simulink model "hip_controller_2026_03_03"  (R2024b)
settings: Solver=FixedStepAuto  StartTime=0.0  StopTime=simDuration  FixedStep=0.01  RelTol=1e-3  EnableMultiTasking=on
InitFcn:
  | breakp=[-1, -0.8, -0.6, -0.4, -0.2, -0.1, 0, 0.1, 0.2, 0.4, 0.6, 0.8, 1];
  | splinenew =[-1, -0.8, -0.6, -0.4, -0.2, -0.1, 0, 0, 0.005, 0.01, 0.015,0.02,0.025];
undefined symbols (not defined in the file or in its folder): Discrete, K, qbreak, Time
libraries: simulink x121, arduinolib x41, dspswit3 x21, ctrlSharedLib x2, dspfdesign x2, slpidlib x2
(part 2 of 7)

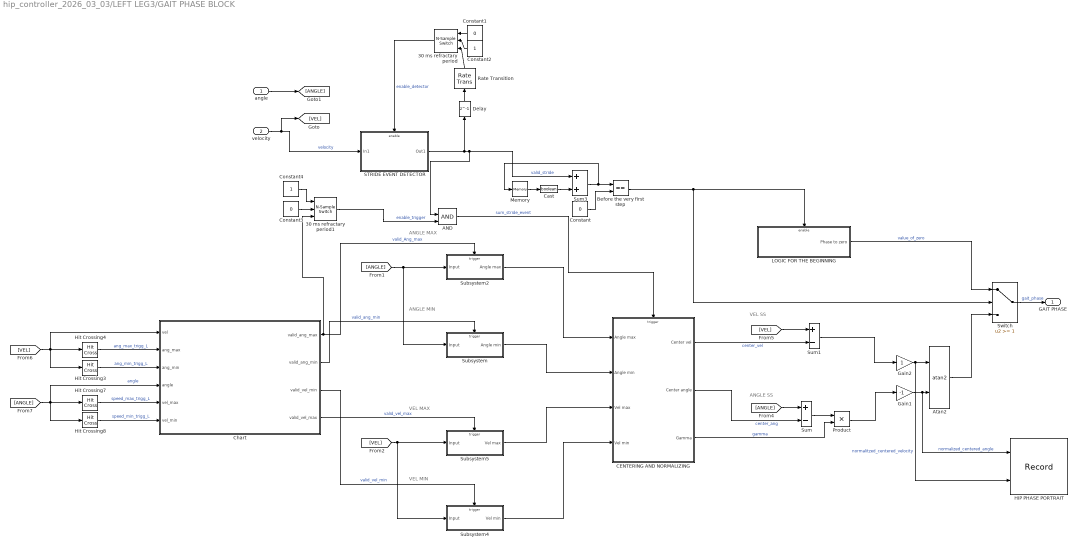
== system hip_controller_2026_03_03/LEFT LEG3/GAIT PHASE BLOCK ==
  note: VEL SS
  note: ANGLE SS
  note: VEL MAX
  note: VEL MIN
  note: ANGLE MIN
  note: ANGLE MAX
  angle : Inport
  velocity : Inport  Port=2
  30 ms refractary period : dspswit3/N-Sample Switch  N=30  reset=on  TriggerType=Rising edge  Ts=-1
  30 ms refractary period1 : dspswit3/N-Sample Switch  N=31  reset=on  TriggerType=Rising edge  Ts=0.01
  AND : Logic  IconShape=distinctive  AllPortsSameDT=off  OutDataTypeStr=boolean
  Atan2 : Trigonometry  Operator=atan2  NumberOfIterations=5
  Before the very first step : RelationalOperator  Operator===  OutDataTypeStr=boolean  RndMeth=Simplest  InputSameDT=off
  CENTERING AND NORMALIZING : Subsystem
  Cast : DataTypeConversion  OutDataTypeStr=boolean  SaturateOnIntegerOverflow=off  RndMeth=Floor
  Chart : Stateflow chart  TreatAsAtomicUnit=on
      settings: PortSchema="{\"entries\":[{\"content\":{\"sides\":[{\"content\":{\"connectorIds\":[\"In5\",\"In1\",\"In4\",\"In6\",\"In3\",\"In2\"]},\"type\":\"ConnectorPlacement.EquallySpacedRectSide\",\"uuid\":\"1b4e9464-0c1b-4aef-9691-eb83c0a92a72\"},{\"content\":{\"connectorIds\":[\"Out3\",\"Out4\",\"Out2\",\"Out1\"],\"side\":\"RIGHT\"},\"type\":\"ConnectorPlacement.EquallySpacedRectSide\",\"uuid\":\"791196f6-4c97-40a1-8015-a03f83b94293\"},{\"content\":{\"side\":\"TOP\"},\"type\":\"ConnectorPlacement.EquallySpacedRectSide\",\"uuid\":\"116d3fb6-be2c-4be4-86cc-df9779b501c6\"}]},\"type\":\"ConnectorPlacement.EquallySpacedConnector\",\"uuid\":\"13d090b2-a2d1-429a-b321-7320a6f027c7\"}],\"packageUris\":[\"http://schema.mathworks.com/mf0/Connector/R2020b\"],\"version\":\"1.0\"}"
  Constant : Constant  Value=0
  Constant1 : Constant  Value=0
  Constant2 : Constant
  Constant3 : Constant  Value=0
  Constant4 : Constant
  Delay : Delay  DelayLength=1
  Gain1 : Gain  Gain=-1
  Gain2 : Gain
  HIP PHASE PORTRAIT : Record  FileSettingsInternal="{\"entries\":[{\"content\":{\"excelSettings\":{\"content\":{},\"type\":\"Streamout.ExcelSettings\"}},\"type\":\"Streamout.FileSettingStorage\",\"uuid\":\"\"}],\"packageUris\":[\"http:\\/\\/schema.mathworks.com\\/mf0\\/streamout_blocks\\/R2020a\"],\"version\":\"1.0\"}"  Layout=[1 1]  SignalsInternal="{\"entries\":[{\"content\":{\"signals\":[{\"content\":{\"blockPath\":[],\"dimensions\":[1],\"domain\":\"\",\"lineColor\":\"#edb120\",\"lineWidth\":2,\"port\":1,\"sid\":[\"\"],\"signalID\":1,\"signalName\":\"normalized_centered_angle\"},\"type\":\"RecordBlkView.Signal\",\"uuid\":\"\"},{\"content\":{\"blockPath\":[],\"dimensions\":[1],\"domain\":\"\",\"lineColor\":\"#7e2f8e\",\"lineWidth\":2,\"port\":2,\"sid\":[\"\"],\"signalID\":2,\"signalName\":\"normalitzed_centered_velocity\"},\"type\":\"RecordBlkView.Signal\",\"uuid\":\"\"}]},\"type\":\"RecordBlkView.InputSignals\",\"uuid\":\"\"}],\"packageUris\":[\"http:\\/\\/schema.mathworks.com\\/mf0\\/streamout_blocks\\/R2020a\"],\"version\":\"1.0\"}"  VisualizationBindings="{\"xyplotplugin\":{\"info\":[{\"series\":[],\"subplotID\":1}]}}"  CompatibilityTag=XY
  Hit Crossing3 : HitCross  HitCrossingDirection=rising
  Hit Crossing4 : HitCross  HitCrossingDirection=falling
  Hit Crossing7 : HitCross  HitCrossingDirection=rising
  Hit Crossing8 : HitCross  HitCrossingDirection=falling
  LOGIC FOR THE BEGINNING : Subsystem
  Memory : Memory
  Product : Product
  Rate Transition : RateTransition  OutPortSampleTime=0.01
  STRIDE EVENT DETECTOR : Subsystem
  Subsystem : Subsystem
  Subsystem2 : Subsystem
  Subsystem4 : Subsystem
  Subsystem5 : Subsystem
  Sum : Sum  Inputs=+-
  Sum1 : Sum  Inputs=+-
  Sum3 : Sum
  Switch : Switch  Threshold=1  SaturateOnIntegerOverflow=off  InputSameDT=off
  GAIT PHASE : Outport
  wires:
  AND/1 -> CENTERING AND NORMALIZING/Trigger  "sum_stride_event"
  Constant4/1 -> 30 ms refractary period1/1
  30 ms refractary period1/1 -> AND/2  "enable_trigger"
  Constant3/1 -> 30 ms refractary period1/2
  Chart/3(valid_ang_max) -> Subsystem2/Trigger, 30 ms refractary period1/3  "valid_Ang_max"
  Chart/1(valid_vel_max) -> Subsystem5/Trigger  "valid_vel_max"
  Chart/2(valid_vel_min) -> Subsystem4/Trigger  "valid_vel_min"
  Chart/4(valid_ang_min) -> Subsystem/Trigger  "valid_ang_min"
  Hit Crossing8/1 -> Chart/2(vel_min)  "speed_min_trigg_L"
  Hit Crossing7/1 -> Chart/3(vel_max)  "speed_max_trigg_L"
  [ANGLE] -> Hit Crossing7/1, Hit Crossing8/1, Chart/6(angle)  "angle"
  Hit Crossing4/1 -> Chart/1(ang_max)  "ang_max_trigg_L"
  Hit Crossing3/1 -> Chart/4(ang_min)  "ang_min_trigg_L"
  [VEL] -> Hit Crossing4/1, Hit Crossing3/1, Chart/5(vel)
  Rate Transition/1 -> 30 ms refractary period/3
  Gain2/1 -> Atan2/1, HIP PHASE PORTRAIT/2  "normalitzed_centered_velocity"
  Delay/1 -> Rate Transition/1
  Constant2/1 -> 30 ms refractary period/2
  Constant1/1 -> 30 ms refractary period/1
  30 ms refractary period/1 -> STRIDE EVENT DETECTOR/Enable  "enable_detector"
  Cast/1 -> Sum3/2
  Memory/1 -> Cast/1
  Switch/1 -> GAIT PHASE/1  "gait_phase"
  LOGIC FOR THE BEGINNING/1(Phase to zero) -> Switch/1  "value_of_zero"
  Before the very first step/1 -> LOGIC FOR THE BEGINNING/Enable, Switch/2
  Constant/1 -> Before the very first step/2
  Sum3/1 -> Before the very first step/1, Memory/1
  Gain1/1 -> Atan2/2, HIP PHASE PORTRAIT/1  "normalized_centered_angle"
  Atan2/1 -> Switch/3
  Sum1/1 -> Gain2/1
  CENTERING AND NORMALIZING/1(Center vel) -> Sum1/2  "center_vel"
  [VEL] -> Sum1/1
  Product/1 -> Gain1/1
  CENTERING AND NORMALIZING/3(Gamma) -> Product/2  "gamma"
  Sum/1 -> Product/1
  CENTERING AND NORMALIZING/2(Center angle) -> Sum/2  "center_ang"
  [ANGLE] -> Sum/1
  Subsystem4/1(Vel min) -> CENTERING AND NORMALIZING/4(Vel min)
  Subsystem5/1(Vel max) -> CENTERING AND NORMALIZING/3(Vel max)
  Subsystem/1(Angle min) -> CENTERING AND NORMALIZING/2(Angle min)
  Subsystem2/1(Angle max) -> CENTERING AND NORMALIZING/1(Angle max)
  STRIDE EVENT DETECTOR/1(Out1) -> Sum3/1, AND/1, Delay/1  "valid_stride"
  [VEL] -> Subsystem5/1(Input), Subsystem4/1(Input)
  [ANGLE] -> Subsystem2/1(Input), Subsystem/1(Input)
  velocity/1 -> [VEL], STRIDE EVENT DETECTOR/1(In1)  "velocity"
  angle/1 -> [ANGLE]

== system hip_controller_2026_03_03/LEFT LEG3/MOTOR POSITION REFERENCE GENERATOR ==
  note: KALMAN FILTER
  GAIT PHASE : Inport
  LAG COMPENSATION : Inport  Port=2
  AMPLITUDE : Inport  Port=3
  Gain : Gain  Gain=-1
  Lookup with Akima spline Interpolation : Lookup_n-D  NumberOfTableDimensions=1  BreakpointsForDimension1=[-5:5]  Table=tanh([-5:5])  InterpMethod=Akima spline  InternalRulePriority=Speed  RndMeth=Simplest
  Motion mapping2 : Lookup_n-D  NumberOfTableDimensions=1  BreakpointsForDimension1=[-1, -0.8, -0.6, -0.4, -0.2, -0.1, 0, 0.1, 0.2, 0.4, 0.6, 0.8, 1]  BreakpointsForDimension2=qbreak(:,2)  Table=[-1, -0.8, -0.6, -0.4, -0.2, -0.1, 0, 0, 0.005, 0.01, 0.015,0.02,0.025]  InterpMethod=Cubic spline  ExtrapMethod=Cubic spline  InternalRulePriority=Speed  RndMeth=Simplest
  Plus : Sum
  Product : Product
  Product1 : Product
  Rate Transition : RateTransition  OutPortSampleTime=0.01
  Ref traj w/ noise : ctrlSharedLib/Kalman Filter  Commented=on  TimeDomain=Discrete-Time  UseCurrentEstimator=off  ModelSource=Individual A, B, C, D matrices  ModelSourceVariable=ss(0.95,1,1,0,1)  A=[1]  B=1  C=[1]  D=0  NumberOfStates=1  NumberOfInputs=1  NumberOfOutputs=1  InitialEstimateSource=Dialog  X0=[0]  P0=10  UseK=off  UseGH=off  NumberOfProcessNoiseInputs=1  G=1  TimeInvariantG=on  H=0  TimeInvariantH=on  Q=1e-3  TimeInvariantQ=on  R=9e-4  TimeInvariantR=on  N=0  TimeInvariantN=on  AddInputPort=off  AddEnablePort=off  OutputEstimatedY=off  OutputP=off  Ts=-1
  Saturation : Saturate  UpperLimit=600*pi/180  LowerLimit=-600*pi/180
  Sin1 : Trigonometry
  Ref motion : Outport
  wires:
  Rate Transition/1 -> Motion mapping2/1  "motion_mapping_key"
  Saturation/1 -> Ref motion/1  "reference_motion"
  Gain/1 -> Rate Transition/1  "left_sin_wave"
  AMPLITUDE/1 -> Product/2  "amplitude"
  LAG COMPENSATION/1 -> Plus/2
  GAIT PHASE/1 -> Plus/1  "gait_phase_left"
  Plus/1 -> Sin1/1
  Sin1/1 -> Gain/1
  Product/1 -> Saturation/1
  Motion mapping2/1 -> Product/1  "motion_mapping_value"
  ? -> Product1/2
  ? -> Product1/1  "motion_mapping_value"

== system hip_controller_2026_03_03/LEFT LEG3/Subsystem ==
  Angle estimation : Inport
  Velocity surrogate (quarature component) : Inport  Port=2
  classif : Inport  Port=3
  Ref amplitude : Inport  Port=4
  sig_power : Inport  Port=5
  Cast To Double : DataTypeConversion  OutDataTypeStr=double  SaturateOnIntegerOverflow=off  RndMeth=Floor
  Chart1 : Stateflow chart  TreatAsAtomicUnit=on
  Constant : Constant
  Product : Product
  Product1 : Product
  SIGMOID SCALING : Subsystem
  Sqrt : Sqrt
  Square : Math  Operator=square
  Square1 : Math  Operator=square
  Sum : Sum
  AMPLITUDE : Outport
  wires:
  Constant/1 -> Chart1/4(Scale_LM)
  Chart1/1(scale) -> Product1/2  "scale=1"
  Product1/1 -> SIGMOID SCALING/1(PORTRAIT RADIUS)
  Angle estimation/1 -> Square/1
  Ref amplitude/1 -> Chart1/2(amplitude)
  sig_power/1 -> Chart1/3(sig_power)
  Velocity surrogate (quarature component)/1 -> Square1/1
  Chart1/2(gain) -> Product/2  "gain=amplitude=6.5"
  Chart1/3(sigmoid_power) -> SIGMOID SCALING/2(Sigmoid Power)  "sigmoid_power=50"
  classif/1 -> Cast To Double/1
  Cast To Double/1 -> Chart1/1(class)
  SIGMOID SCALING/1(Out1) -> Product/1
  Sqrt/1 -> Product1/1  "PORTRAIT RADIUS"
  Product/1 -> AMPLITUDE/1
  Sum/1 -> Sqrt/1
  Square1/1 -> Sum/2
  Square/1 -> Sum/1

== system hip_controller_2026_03_03/Prerecorded Data/Subsystem1 ==
  x : Inport
  Constant : Constant  Value=2
  Integrator1 : Integrator  InitialConditionSource=external
  Integrator2 : Integrator
  Product : Product  RndMeth=Zero
  Product1 : Product  RndMeth=Zero
  Product2 : Product  Inputs=3  RndMeth=Zero
  Sum : Sum  Inputs=|+-
  Sum1 : Sum  Inputs=|+-
  wn : Constant  Value=wn
  x0 : Constant  Value=x0
  zt : Constant  Value=zt
  y : Outport  VectorParamsAs1DForOutWhenUnconnected=off
  wires:
  Sum/1 -> Product/2
  wn/1 -> Product/1, Product1/1
  Sum1/1 -> Sum/1
  x0/1 -> Integrator1/2
  Integrator2/1 -> Product1/2, Product2/1
  Product/1 -> Integrator2/1
  x/1 -> Sum1/1
  Product1/1 -> Integrator1/1
  Integrator1/1 -> Sum1/2, y/1
  Product2/1 -> Sum/2
  zt/1 -> Product2/3
  Constant/1 -> Product2/2

== system hip_controller_2026_03_03/Prerecorded Data/Subsystem2 ==
  x : Inport
  Constant : Constant  Value=2
  Integrator1 : Integrator  InitialConditionSource=external
  Integrator2 : Integrator
  Product : Product  RndMeth=Zero
  Product1 : Product  RndMeth=Zero
  Product2 : Product  Inputs=3  RndMeth=Zero
  Sum : Sum  Inputs=|+-
  Sum1 : Sum  Inputs=|+-
  wn : Constant  Value=wn
  x0 : Constant  Value=x0
  zt : Constant  Value=zt
  y : Outport  VectorParamsAs1DForOutWhenUnconnected=off
  yd : Outport  Port=2
  wires:
  Sum/1 -> Product/2  "e2=e1-feedback"
  wn/1 -> Product/1, Product1/1  "wn"
  Sum1/1 -> Sum/1  "e1=x-y"
  x0/1 -> Integrator1/2  "x0=0"
  Integrator2/1 -> Product2/1, Product1/2  "integrator(wn*e2)"
  Product/1 -> Integrator2/1  "wn*e2"
  x/1 -> Sum1/1  "x"
  Product1/1 -> Integrator1/1, yd/1  "yd"
  Integrator1/1 -> Sum1/2, y/1  "y"
  Product2/1 -> Sum/2  "feedback"
  zt/1 -> Product2/3  "zt=1"
  Constant/1 -> Product2/2

== system hip_controller_2026_03_03/Prerecorded Data/Subsystem3 ==
  x : Inport
  Constant : Constant  Value=2
  Integrator1 : Integrator  InitialConditionSource=external
  Integrator2 : Integrator
  Product : Product  RndMeth=Zero
  Product1 : Product  RndMeth=Zero
  Product2 : Product  Inputs=3  RndMeth=Zero
  Sum : Sum  Inputs=|+-
  Sum1 : Sum  Inputs=|+-
  wn : Constant  Value=wn
  x0 : Constant  Value=x0
  zt : Constant  Value=zt
  y : Outport  VectorParamsAs1DForOutWhenUnconnected=off
  wires:
  Sum/1 -> Product/2
  wn/1 -> Product/1, Product1/1
  Sum1/1 -> Sum/1
  x0/1 -> Integrator1/2
  Integrator2/1 -> Product1/2, Product2/1
  Product/1 -> Integrator2/1
  x/1 -> Sum1/1
  Product1/1 -> Integrator1/1
  Integrator1/1 -> Sum1/2, y/1
  Product2/1 -> Sum/2
  zt/1 -> Product2/3
  Constant/1 -> Product2/2

== system hip_controller_2026_03_03/Prerecorded Data/Subsystem4 ==
  x : Inport
  Constant : Constant  Value=2
  Integrator1 : Integrator  InitialConditionSource=external
  Integrator2 : Integrator
  Product : Product  RndMeth=Zero
  Product1 : Product  RndMeth=Zero
  Product2 : Product  Inputs=3  RndMeth=Zero
  Sum : Sum  Inputs=|+-
  Sum1 : Sum  Inputs=|+-
  wn : Constant  Value=wn
  x0 : Constant  Value=x0
  zt : Constant  Value=zt
  y : Outport  VectorParamsAs1DForOutWhenUnconnected=off
  wires:
  Sum/1 -> Product/2
  wn/1 -> Product/1, Product1/1
  Sum1/1 -> Sum/1
  x0/1 -> Integrator1/2
  Integrator2/1 -> Product1/2, Product2/1
  Product/1 -> Integrator2/1
  x/1 -> Sum1/1
  Product1/1 -> Integrator1/1
  Integrator1/1 -> Sum1/2, y/1
  Product2/1 -> Sum/2
  zt/1 -> Product2/3
  Constant/1 -> Product2/2

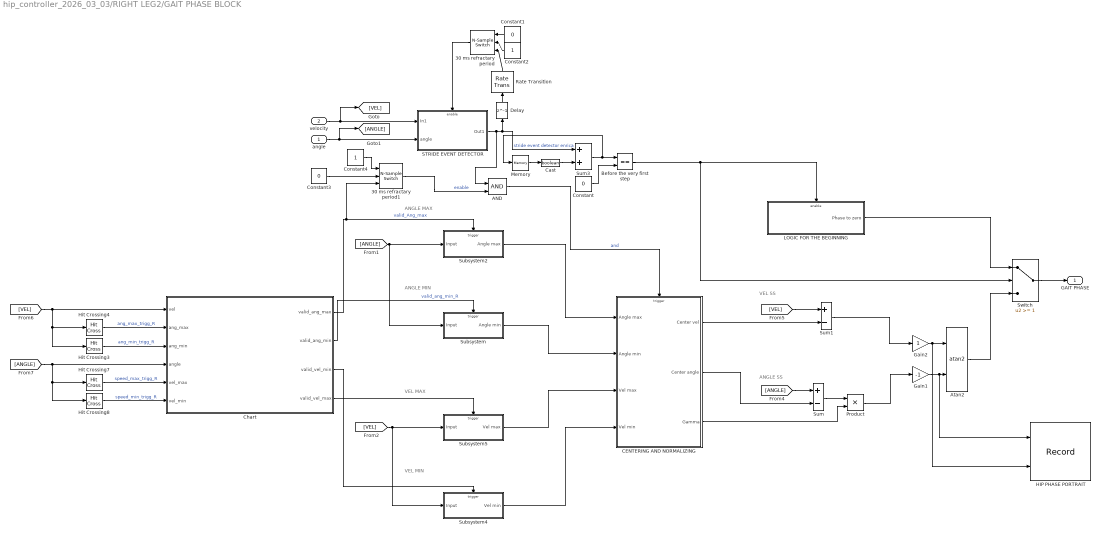
== system hip_controller_2026_03_03/RIGHT LEG2/GAIT PHASE BLOCK ==
  note: VEL SS
  note: ANGLE SS
  note: VEL MAX
  note: VEL MIN
  note: ANGLE MIN
  note: ANGLE MAX
  angle : Inport
  velocity : Inport  Port=2
  30 ms refractary period : dspswit3/N-Sample Switch  N=30  reset=on  TriggerType=Rising edge  Ts=-1
  30 ms refractary period1 : dspswit3/N-Sample Switch  N=31  reset=on  TriggerType=Rising edge  Ts=0.01
  AND : Logic  IconShape=distinctive  AllPortsSameDT=off  OutDataTypeStr=boolean
  Atan2 : Trigonometry  Operator=atan2  NumberOfIterations=5
  Before the very first step : RelationalOperator  Operator===  OutDataTypeStr=boolean  RndMeth=Simplest  InputSameDT=off
  CENTERING AND NORMALIZING : Subsystem
  Cast : DataTypeConversion  OutDataTypeStr=boolean  SaturateOnIntegerOverflow=off  RndMeth=Floor
  Chart : Stateflow chart  TreatAsAtomicUnit=on
      settings: PortSchema="{\"entries\":[{\"content\":{\"sides\":[{\"content\":{\"connectorIds\":[\"In5\",\"In1\",\"In4\",\"In6\",\"In3\",\"In2\"]},\"type\":\"ConnectorPlacement.EquallySpacedRectSide\",\"uuid\":\"1b4e9464-0c1b-4aef-9691-eb83c0a92a72\"},{\"content\":{\"connectorIds\":[\"Out3\",\"Out4\",\"Out2\",\"Out1\"],\"side\":\"RIGHT\"},\"type\":\"ConnectorPlacement.EquallySpacedRectSide\",\"uuid\":\"791196f6-4c97-40a1-8015-a03f83b94293\"},{\"content\":{\"side\":\"TOP\"},\"type\":\"ConnectorPlacement.EquallySpacedRectSide\",\"uuid\":\"116d3fb6-be2c-4be4-86cc-df9779b501c6\"}]},\"type\":\"ConnectorPlacement.EquallySpacedConnector\",\"uuid\":\"13d090b2-a2d1-429a-b321-7320a6f027c7\"}],\"packageUris\":[\"http://schema.mathworks.com/mf0/Connector/R2020b\"],\"version\":\"1.0\"}"
  Constant : Constant  Value=0
  Constant1 : Constant  Value=0
  Constant2 : Constant
  Constant3 : Constant  Value=0
  Constant4 : Constant
  Delay : Delay  DelayLength=1
  Gain1 : Gain  Gain=-1
  Gain2 : Gain
  HIP PHASE PORTRAIT : Record  FileSettingsInternal="{\"entries\":[{\"content\":{\"excelSettings\":{\"content\":{},\"type\":\"Streamout.ExcelSettings\"}},\"type\":\"Streamout.FileSettingStorage\",\"uuid\":\"\"}],\"packageUris\":[\"http:\\/\\/schema.mathworks.com\\/mf0\\/streamout_blocks\\/R2020a\"],\"version\":\"1.0\"}"  Layout=[1 1]  SignalsInternal="{\"entries\":[{\"content\":{\"signals\":[{\"content\":{\"blockPath\":[],\"dimensions\":[1],\"domain\":\"\",\"lineColor\":\"#ff6929\",\"lineWidth\":2,\"port\":1,\"sid\":[\"\"],\"signalID\":1,\"signalName\":\"Gain1\"},\"type\":\"RecordBlkView.Signal\",\"uuid\":\"\"},{\"content\":{\"blockPath\":[],\"dimensions\":[1],\"domain\":\"\",\"lineColor\":\"#b746ff\",\"lineWidth\":2,\"port\":2,\"sid\":[\"\"],\"signalID\":2,\"signalName\":\"Gain2\"},\"type\":\"RecordBlkView.Signal\",\"uuid\":\"\"}]},\"type\":\"RecordBlkView.InputSignals\",\"uuid\":\"\"}],\"packageUris\":[\"http:\\/\\/schema.mathworks.com\\/mf0\\/streamout_blocks\\/R2020a\"],\"version\":\"1.0\"}"  VisualizationBindings="{\"xyplotplugin\":{\"info\":[{\"series\":[],\"subplotID\":1}]}}"  CompatibilityTag=XY
  Hit Crossing3 : HitCross  HitCrossingDirection=rising
  Hit Crossing4 : HitCross  HitCrossingDirection=falling
  Hit Crossing7 : HitCross  HitCrossingDirection=rising
  Hit Crossing8 : HitCross  HitCrossingDirection=falling
  LOGIC FOR THE BEGINNING : Subsystem
  Memory : Memory
  Product : Product
  Rate Transition : RateTransition  OutPortSampleTime=0.01
  STRIDE EVENT DETECTOR : Subsystem
  Subsystem : Subsystem
  Subsystem2 : Subsystem
  Subsystem4 : Subsystem
  Subsystem5 : Subsystem
  Sum : Sum  Inputs=+-
  Sum1 : Sum  Inputs=+-
  Sum3 : Sum
  Switch : Switch  Threshold=1  SaturateOnIntegerOverflow=off  InputSameDT=off
  GAIT PHASE : Outport
  wires:
  AND/1 -> CENTERING AND NORMALIZING/Trigger  "and"
  Constant4/1 -> 30 ms refractary period1/1
  STRIDE EVENT DETECTOR/1(Out1) -> Sum3/1, Delay/1, AND/1  "stride event detector enrica"
  30 ms refractary period1/1 -> AND/2  "enable"
  Constant3/1 -> 30 ms refractary period1/2
  Chart/3(valid_ang_max) -> 30 ms refractary period1/3, Subsystem2/Trigger  "valid_Ang_max"
  Chart/1(valid_vel_max) -> Subsystem5/Trigger
  Chart/4(valid_ang_min) -> Subsystem/Trigger  "valid_ang_min_R"
  Hit Crossing8/1 -> Chart/2(vel_min)  "speed_min_trigg_R"
  Hit Crossing4/1 -> Chart/1(ang_max)  "ang_max_trigg_R"
  [ANGLE] -> Chart/6(angle), Hit Crossing7/1, Hit Crossing8/1
  Hit Crossing7/1 -> Chart/3(vel_max)  "speed_max_trigg_R"
  [VEL] -> Chart/5(vel), Hit Crossing4/1, Hit Crossing3/1
  Hit Crossing3/1 -> Chart/4(ang_min)  "ang_min_trigg_R"
  Rate Transition/1 -> 30 ms refractary period/3
  Gain2/1 -> Atan2/1, HIP PHASE PORTRAIT/2
  Delay/1 -> Rate Transition/1
  Constant2/1 -> 30 ms refractary period/2
  Constant1/1 -> 30 ms refractary period/1
  30 ms refractary period/1 -> STRIDE EVENT DETECTOR/Enable
  Cast/1 -> Sum3/2
  Memory/1 -> Cast/1
  Switch/1 -> GAIT PHASE/1
  LOGIC FOR THE BEGINNING/1(Phase to zero) -> Switch/1
  Before the very first step/1 -> LOGIC FOR THE BEGINNING/Enable, Switch/2
  Constant/1 -> Before the very first step/2
  Sum3/1 -> Before the very first step/1, Memory/1
  Gain1/1 -> Atan2/2, HIP PHASE PORTRAIT/1
  Atan2/1 -> Switch/3
  Sum1/1 -> Gain2/1
  CENTERING AND NORMALIZING/1(Center vel) -> Sum1/2
  [VEL] -> Sum1/1
  Product/1 -> Gain1/1
  CENTERING AND NORMALIZING/3(Gamma) -> Product/2
  Sum/1 -> Product/1
  CENTERING AND NORMALIZING/2(Center angle) -> Sum/2
  [ANGLE] -> Sum/1
  Subsystem4/1(Vel min) -> CENTERING AND NORMALIZING/4(Vel min)
  Subsystem5/1(Vel max) -> CENTERING AND NORMALIZING/3(Vel max)
  Subsystem/1(Angle min) -> CENTERING AND NORMALIZING/2(Angle min)
  Subsystem2/1(Angle max) -> CENTERING AND NORMALIZING/1(Angle max)
  [VEL] -> Subsystem5/1(Input), Subsystem4/1(Input)
  Chart/2(valid_vel_min) -> Subsystem4/Trigger
  [ANGLE] -> Subsystem2/1(Input), Subsystem/1(Input)
  velocity/1 -> [VEL], STRIDE EVENT DETECTOR/1(In1)
  angle/1 -> STRIDE EVENT DETECTOR/2(angle), [ANGLE]

== system hip_controller_2026_03_03/RIGHT LEG2/MOTOR POSITION REFERENCE GENERATOR ==
  note: KALMAN FILTER
  GAIT PHASE : Inport
  LAG COMPENSATION : Inport  Port=2
  AMPLITUDE : Inport  Port=3
  Gain : Gain  Gain=-1
  Motion mapping2 : Lookup_n-D  NumberOfTableDimensions=1  BreakpointsForDimension1=[-1, -0.8, -0.6, -0.4, -0.2, -0.1, 0, 0.1, 0.2, 0.4, 0.6, 0.8, 1]  BreakpointsForDimension2=qbreak(:,2)  Table=[-1, -0.8, -0.6, -0.4, -0.2, -0.1, 0, 0, 0.005, 0.01, 0.015,0.02,0.025]  InterpMethod=Cubic spline  ExtrapMethod=Cubic spline  InternalRulePriority=Speed  RndMeth=Simplest
  Plus : Sum
  Product : Product
  Rate Transition : RateTransition  OutPortSampleTime=0.01
  Ref traj w/ noise : ctrlSharedLib/Kalman Filter  Commented=on  TimeDomain=Discrete-Time  UseCurrentEstimator=off  ModelSource=Individual A, B, C, D matrices  ModelSourceVariable=ss(0.95,1,1,0,1)  A=[1]  B=1  C=[1]  D=0  NumberOfStates=1  NumberOfInputs=1  NumberOfOutputs=1  InitialEstimateSource=Dialog  X0=[0]  P0=10  UseK=off  UseGH=off  NumberOfProcessNoiseInputs=1  G=1  TimeInvariantG=on  H=0  TimeInvariantH=on  Q=1e-3  TimeInvariantQ=on  R=9e-4  TimeInvariantR=on  N=0  TimeInvariantN=on  AddInputPort=off  AddEnablePort=off  OutputEstimatedY=off  OutputP=off  Ts=-1
  Saturation : Saturate  UpperLimit=600*pi/180  LowerLimit=-600*pi/180
  Sin1 : Trigonometry
  Ref motion : Outport
  wires:
  Rate Transition/1 -> Motion mapping2/1  "right_sin_wave"
  Saturation/1 -> Ref motion/1  "ref_motion"
  Gain/1 -> Rate Transition/1  "sin_wave"
  AMPLITUDE/1 -> Product/2  "amplitude"
  LAG COMPENSATION/1 -> Plus/2
  GAIT PHASE/1 -> Plus/1  "gait_phase"
  Plus/1 -> Sin1/1
  Sin1/1 -> Gain/1
  Product/1 -> Saturation/1
  Motion mapping2/1 -> Product/1

== system hip_controller_2026_03_03/RIGHT LEG2/Subsystem ==
  Angle estimation : Inport
  Velocity surrogate (quarature component) : Inport  Port=2
  Ref amplitude : Inport  Port=3
  classif : Inport  Port=4
  Sig_Power : Inport  Port=5
  Cast To Double : DataTypeConversion  OutDataTypeStr=double  SaturateOnIntegerOverflow=off  RndMeth=Floor
  Chart1 : Stateflow chart  TreatAsAtomicUnit=on
  Constant : Constant
  Product : Product
  Product1 : Product
  SIGMOID SCALING : Subsystem
  Sqrt : Sqrt
  Square : Math  Operator=square
  Square1 : Math  Operator=square
  Sum : Sum
  Amplitude_R : Outport
  wires:
  Chart1/1(scale_LM) -> Product1/2
  Constant/1 -> Chart1/4("scale_LM "), Chart1/5(Scale)
  Product1/1 -> SIGMOID SCALING/1(PORTRAIT RADIUS)
  Angle estimation/1 -> Square/1
  Sig_Power/1 -> Chart1/3(sig_power)
  Velocity surrogate (quarature component)/1 -> Square1/1
  Chart1/2(gain) -> Product/2
  Sqrt/1 -> Product1/1  "PORTRAIT RADIUS R"
  Chart1/3(sigmoid_power) -> SIGMOID SCALING/2(sigmoid_power)
  Ref amplitude/1 -> Chart1/2(amplitude)
  classif/1 -> Cast To Double/1
  Cast To Double/1 -> Chart1/1(class)
  SIGMOID SCALING/1(Out1) -> Product/1  "Sig_Scale_R"
  Product/1 -> Amplitude_R/1
  Sum/1 -> Sqrt/1
  Square1/1 -> Sum/2
  Square/1 -> Sum/1

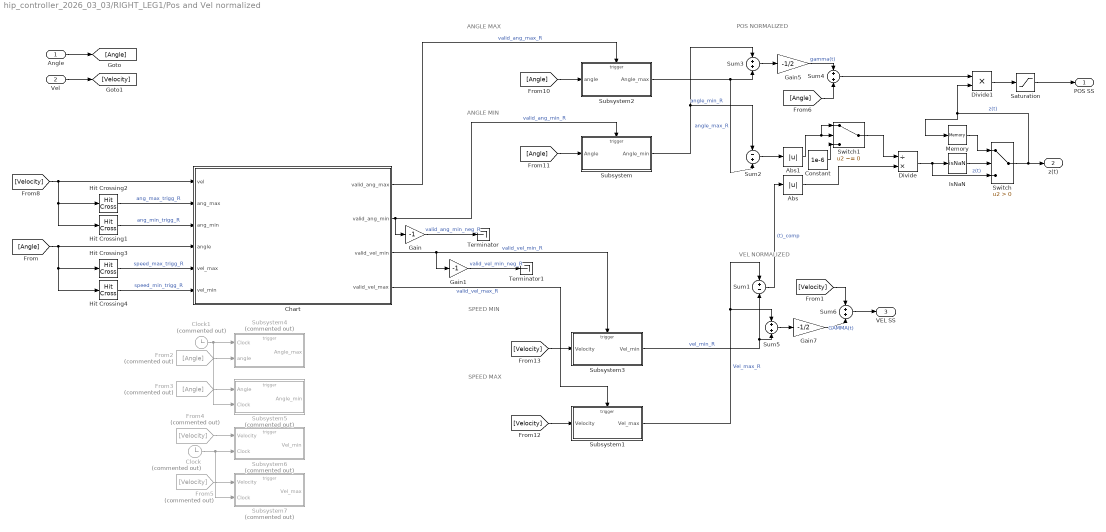
== system hip_controller_2026_03_03/RIGHT_LEG1/Pos and Vel normalized ==
  note: ANGLE MIN
  note: ANGLE MAX
  note: SPEED MAX
  note: SPEED MIN
  note: POS NORMALIZED
  note: VEL NORMALIZED
  Angle : Inport
  Vel : Inport  Port=2
  Abs : Abs  SaturateOnIntegerOverflow=off
  Abs1 : Abs  SaturateOnIntegerOverflow=off
  Chart : Stateflow chart  TreatAsAtomicUnit=on
      settings: PortSchema="{\"entries\":[{\"content\":{\"sides\":[{\"content\":{\"connectorIds\":[\"In5\",\"In1\",\"In4\",\"In6\",\"In3\",\"In2\"]},\"type\":\"ConnectorPlacement.EquallySpacedRectSide\",\"uuid\":\"1b4e9464-0c1b-4aef-9691-eb83c0a92a72\"},{\"content\":{\"connectorIds\":[\"Out3\",\"Out4\",\"Out2\",\"Out1\"],\"side\":\"RIGHT\"},\"type\":\"ConnectorPlacement.EquallySpacedRectSide\",\"uuid\":\"791196f6-4c97-40a1-8015-a03f83b94293\"},{\"content\":{\"side\":\"TOP\"},\"type\":\"ConnectorPlacement.EquallySpacedRectSide\",\"uuid\":\"116d3fb6-be2c-4be4-86cc-df9779b501c6\"}]},\"type\":\"ConnectorPlacement.EquallySpacedConnector\",\"uuid\":\"13d090b2-a2d1-429a-b321-7320a6f027c7\"}],\"packageUris\":[\"http://schema.mathworks.com/mf0/Connector/R2020b\"],\"version\":\"1.0\"}"
  Clock : Clock  Commented=on
  Clock1 : Clock  Commented=on
  Constant : Constant  Value=1e-6
  Divide : Product  Inputs=/*
  Divide1 : Product  Inputs=**
  From2 : From  Commented=on  GotoTag=Angle
  From3 : From  Commented=on  GotoTag=Angle
  From4 : From  Commented=on  GotoTag=Velocity
  From5 : From  Commented=on  GotoTag=Velocity
  Gain : Gain  Gain=-1
  Gain1 : Gain  Gain=-1
  Gain5 : Gain  Gain=-1/2
  Gain7 : Gain  Gain=-1/2
  Hit Crossing1 : HitCross  HitCrossingDirection=rising
  Hit Crossing2 : HitCross  HitCrossingDirection=falling
  Hit Crossing3 : HitCross  HitCrossingDirection=rising
  Hit Crossing4 : HitCross  HitCrossingDirection=falling
  IsNaN : RelationalOperator  Operator=isNaN  OutDataTypeStr=boolean  RndMeth=Simplest  InputSameDT=off
  Memory : Memory
  Saturation : Saturate  UpperLimit=10  LowerLimit=-10
  Subsystem : Subsystem
  Subsystem1 : Subsystem
  Subsystem2 : Subsystem
  Subsystem3 : Subsystem
  Subsystem4 : Subsystem  Commented=on
  Subsystem5 : Subsystem  Commented=on
  Subsystem6 : Subsystem  Commented=on
  Subsystem7 : Subsystem  Commented=on
  Sum1 : Sum  Inputs=+-
  Sum2 : Sum  Inputs=-+
  Sum{3..6} (4 alike) : Sum
  Switch : Switch  Criteria=u2 > Threshold  SaturateOnIntegerOverflow=off  InputSameDT=off
  Switch1 : Switch  Criteria=u2 ~= 0  SaturateOnIntegerOverflow=off  InputSameDT=off
  Terminator : Terminator
  Terminator1 : Terminator
  POS SS : Outport
  z(t) : Outport  Port=2
  VEL SS : Outport  Port=3
  wires:
  Hit Crossing2/1 -> Chart/1(ang_max)  "ang_max_trigg_R"
  Subsystem2/1(Angle_max) -> Sum2/2, Sum3/2  "angle_max_R"
  Sum4/1 -> Divide1/1
  Sum3/1 -> Gain5/1
  Subsystem/1(Angle_min) -> Sum2/1, Sum3/1  "angle_min_R"
  Hit Crossing1/1 -> Chart/4(ang_min)  "ang_min_trigg_R"
  Sum2/1 -> Abs1/1
  Sum1/1 -> Abs/1  "(t)_comp"
  Gain5/1 -> Sum4/1  "gamma(t)"
  Abs/1 -> Divide/2
  Divide/1 -> IsNaN/1, Switch/3  "z(t)"
  Memory/1 -> Switch/1
  IsNaN/1 -> Switch/2
  Switch/1 -> Memory/1, Divide1/2, z(t)/1  "z(t)"
  Divide1/1 -> Saturation/1
  Saturation/1 -> POS SS/1
  Clock1/1 -> Subsystem5/2(Clock), Subsystem4/1(Clock)
  Constant/1 -> Switch1/3
  Abs1/1 -> Switch1/2, Switch1/1
  Switch1/1 -> Divide/1
  Clock/1 -> Subsystem7/2(Clock), Subsystem6/2(Clock)
  Hit Crossing4/1 -> Chart/2(vel_min)  "speed_min_trigg_R"
  Subsystem3/1(Vel_min) -> Sum1/2, Sum5/2  "vel_min_R"
  Subsystem1/1(Vel_max) -> Sum1/1, Sum5/1  "Vel_max_R"
  Sum5/1 -> Gain7/1
  Hit Crossing3/1 -> Chart/3(vel_max)  "speed_max_trigg_R"
  Sum6/1 -> VEL SS/1
  Gain7/1 -> Sum6/2  "GAMMA(t)"
  [Velocity] -> Sum6/1
  Chart/1(valid_vel_max) -> Subsystem1/Trigger  "valid_vel_max_R"
  Chart/4(valid_ang_min) -> Gain/1, Subsystem/Trigger  "valid_ang_min_R"
  Chart/3(valid_ang_max) -> Subsystem2/Trigger  "valid_ang_max_R"
  Chart/2(valid_vel_min) -> Gain1/1, Subsystem3/Trigger  "valid_vel_min_R"
  Vel/1 -> [Velocity]
  Angle/1 -> [Angle]
  From5/1 -> Subsystem7/1(Velocity)
  From4/1 -> Subsystem6/1(Velocity)
  From3/1 -> Subsystem5/1(Angle)
  From2/1 -> Subsystem4/2(angle)
  [Angle] -> Hit Crossing4/1, Hit Crossing3/1, Chart/6(angle)
  [Angle] -> Subsystem/1(Angle)
  [Angle] -> Subsystem2/1(angle)
  [Velocity] -> Subsystem1/1(Velocity)
  [Velocity] -> Subsystem3/1(Velocity)
  [Velocity] -> Hit Crossing1/1, Hit Crossing2/1, Chart/5(vel)
  Gain/1 -> Terminator/1  "valid_ang_min_neg_R"
  Gain1/1 -> Terminator1/1  "valid_vel_min_neg_R"
  [Angle] -> Sum4/2

== system hip_controller_2026_03_03/RIGHT_LEG1/STOP CONDITION ==
  position : Inport
  speed : Inport  Port=2
  Constant : Constant
  Constant1 : Constant  Value=0
  Sqrt : Sqrt
  Square : Math  Operator=square
  Square1 : Math  Operator=square
  Sum : Sum
  Switch3 : Switch  Criteria=u2 > Threshold  Threshold=0.3  SaturateOnIntegerOverflow=off  InputSameDT=off
  Check : Outport
  Walking frequency : Outport  Port=2
  wires:
  position/1 -> Square/1  "θ"
  speed/1 -> Square1/1  "θ_dot"
  Square/1 -> Sum/1
  Square1/1 -> Sum/2
  Sum/1 -> Sqrt/1
  Constant/1 -> Switch3/1
  Constant1/1 -> Switch3/3
  Sqrt/1 -> Switch3/2, Walking frequency/1
  Switch3/1 -> Check/1

== system hip_controller_2026_03_03/Subsystem3/Left Motor Velocity ==
  SWITCH : Inport
  Motor command : Inport  Port=2
  Motor Actual Position Receive : Subsystem
  Subsystem : Subsystem
  MOTOR POSITION : Outport
  MOTOR SPEED : Outport  Port=2
  MOTOR TORQUE : Outport  Port=3
  wires:
  Motor command/1 -> Subsystem/1(Motor command)
  SWITCH/1 -> Motor Actual Position Receive/1(SWITCH), Subsystem/2(SWITCH)
  Motor Actual Position Receive/1(MOTOR POSITION) -> MOTOR POSITION/1
  Motor Actual Position Receive/2(MOTOR SPEED) -> MOTOR SPEED/1
  Motor Actual Position Receive/3(MOTOR TORQUE) -> MOTOR TORQUE/1

== system hip_controller_2026_03_03/Subsystem3/Right Motor Velocity ==
  SWITCH : Inport
  Motor command : Inport  Port=2
  Motor Actual Position Receive : Subsystem
  Subsystem : Subsystem
  MOTOR POSITION : Outport
  MOTOR SPEED : Outport  Port=2
  MOTOR TORQUE : Outport  Port=3
  wires:
  Motor command/1 -> Subsystem/1(Motor command)
  SWITCH/1 -> Motor Actual Position Receive/1(SWITCH), Subsystem/2(SWITCH)
  Motor Actual Position Receive/1(MOTOR POSITION) -> MOTOR POSITION/1
  Motor Actual Position Receive/2(MOTOR SPEED) -> MOTOR SPEED/1
  Motor Actual Position Receive/3(MOTOR TORQUE) -> MOTOR TORQUE/1

== system hip_controller_2026_03_03/Subsystem3/Subsystem1 ==
  x : Inport
  Constant : Constant  Value=2
  Integrator1 : Integrator  InitialConditionSource=external
  Integrator2 : Integrator
  Product : Product  RndMeth=Zero
  Product1 : Product  RndMeth=Zero
  Product2 : Product  Inputs=3  RndMeth=Zero
  Sum : Sum  Inputs=|+-
  Sum1 : Sum  Inputs=|+-
  wn : Constant  Value=wn
  x0 : Constant  Value=x0
  zt : Constant  Value=zt
  y : Outport  VectorParamsAs1DForOutWhenUnconnected=off
  yd : Outport  Port=2  VectorParamsAs1DForOutWhenUnconnected=off
  wires:
  Sum/1 -> Product/2
  wn/1 -> Product/1, Product1/1
  Sum1/1 -> Sum/1
  x0/1 -> Integrator1/2
  Integrator2/1 -> Product1/2, Product2/1
  Product/1 -> Integrator2/1
  x/1 -> Sum1/1
  Product1/1 -> Integrator1/1, yd/1
  Integrator1/1 -> Sum1/2, y/1
  Product2/1 -> Sum/2
  zt/1 -> Product2/3
  Constant/1 -> Product2/2

== system hip_controller_2026_03_03/Subsystem3/Subsystem4 ==
  x : Inport
  Constant : Constant  Value=2
  Integrator1 : Integrator  InitialConditionSource=external
  Integrator2 : Integrator
  Product : Product  RndMeth=Zero
  Product1 : Product  RndMeth=Zero
  Product2 : Product  Inputs=3  RndMeth=Zero
  Sum : Sum  Inputs=|+-
  Sum1 : Sum  Inputs=|+-
  wn : Constant  Value=wn
  x0 : Constant  Value=x0
  zt : Constant  Value=zt
  y : Outport  VectorParamsAs1DForOutWhenUnconnected=off
  yd : Outport  Port=2  VectorParamsAs1DForOutWhenUnconnected=off
  wires:
  Sum/1 -> Product/2
  wn/1 -> Product/1, Product1/1
  Sum1/1 -> Sum/1
  x0/1 -> Integrator1/2
  Integrator2/1 -> Product1/2, Product2/1
  Product/1 -> Integrator2/1
  x/1 -> Sum1/1
  Product1/1 -> Integrator1/1, yd/1
  Integrator1/1 -> Sum1/2, y/1
  Product2/1 -> Sum/2
  zt/1 -> Product2/3
  Constant/1 -> Product2/2

== system hip_controller_2026_03_03/Subsystem4/Left Motor Velocity ==
  SWITCH : Inport
  Motor command : Inport  Port=2
  Motor Actual Position Receive : Subsystem
  Subsystem : Subsystem
  MOTOR POSITION : Outport
  MOTOR SPEED : Outport  Port=2
  MOTOR TORQUE : Outport  Port=3
  wires:
  Motor command/1 -> Subsystem/1(Motor command)
  SWITCH/1 -> Motor Actual Position Receive/1(SWITCH), Subsystem/2(SWITCH)
  Motor Actual Position Receive/1(MOTOR POSITION) -> MOTOR POSITION/1
  Motor Actual Position Receive/2(MOTOR SPEED) -> MOTOR SPEED/1
  Motor Actual Position Receive/3(MOTOR TORQUE) -> MOTOR TORQUE/1

== system hip_controller_2026_03_03/Subsystem4/PID1 ==
  Ref : Inport
  Actual Motion : Inport  Port=2
  Enable : EnablePort  StatesWhenEnabling=reset
  PID Controller1 : slpidlib/PID Controller  Controller=PID  Form=Parallel  TimeDomain=Continuous-time  UseExternalTs=off  SampleTime=-1  IntegratorMethod=Forward Euler  FilterMethod=Forward Euler  ControllerParametersSource=internal  P=1  I=1  UseKiTs=off  D=0  N=100  UseFilter=on  TunerSelectOption=Transfer Function Based (PID Tuner App)  InitialConditionSource=internal  InitialConditionForIntegrator=0  InitialConditionForFilter=0  DifferentiatorICPrevScaledInput=0  ExternalReset=none  TrackingMode=off  Kt=1  LimitOutput=off  SatLimitsSource=internal  UpperSaturationLimit=inf  LowerSaturationLimit=-inf  LinearizeAsGain=on  AntiWindupMode=none  Kb=1  LimitIntegrator=off  UpperIntegratorSaturationLimit=inf  LowerIntegratorSaturationLimit=-inf  POutMin=[]  POutMax=[]  IOutMin=[]  IOutMax=[]  DOutMin=[]  DOutMax=[]  NOutMin=[]  NOutMax=[]  SumOutMin=[]  SumOutMax=[]  SaturationOutMin=[]  SaturationOutMax=[]  PParamMin=[]  PParamMax=[]  IParamMin=[]  IParamMax=[]  DParamMin=[]  DParamMax=[]  NParamMin=[]  NParamMax=[]  KbParamMin=[]  KbParamMax=[]  KtParamMin=[]  KtParamMax=[]  KbOutMin=[]  KbOutMax=[]  KtOutMin=[]  KtOutMax=[]  IntegratorOutMin=[]  IntegratorOutMax=[]  FilterOutMin=[]  FilterOutMax=[]  SumI1OutMin=[]  SumI1OutMax=[]  SumI2OutMin=[]  SumI2OutMax=[]  SumI3OutMin=[]  SumI3OutMax=[]  SumI4OutMin=[]  SumI4OutMax=[]  SumDOutMin=[]  SumDOutMax=[]  DifferentiatorOutMin=[]  DifferentiatorOutMax=[]  FilterDiffOutCoefMin=[]  FilterDiffOutCoefMax=[]  ReciprocalOutMin=[]  ReciprocalOutMax=[]  SumDenOutMin=[]  SumDenOutMax=[]  SumNumOutMin=[]  SumNumOutMax=[]  DivideOutMin=[]  DivideOutMax=[]  UdiffTsProdOutMin=[]  UdiffTsProdOutMax=[]  NTsProdOutMin=[]  NTsProdOutMax=[]  UintegralTsProdOutMin=[]  UintegralTsProdOutMax=[]  UngainTsProdOutMin=[]  UngainTsProdOutMax=[]  ClampingZeroOutDataTypeStr=Inherit: Inherit via back propagation  ClampingZeroOutMin=[]  ClampingZeroOutMax=[]  FilterDenConstantOutDataTypeStr=Inherit: Inherit via back propagation  FilterDenConstantOutMin=[]  FilterDenConstantOutMax=[]  PCopyOutDataTypeStr=Inherit: Inherit via back propagation  PCopyOutMin=[]  PCopyOutMax=[]  NCopyOutDataTypeStr=Inherit: Inherit via back propagation  NCopyOutMin=[]  NCopyOutMax=[]  IntegratorContinuousStateAttributes=''  IntegratorStateMustResolveToSignalObject=off  IntegratorRTWStateStorageClass=Auto  FilterContinuousStateAttributes=''  FilterStateMustResolveToSignalObject=off  FilterRTWStateStorageClass=Auto  ParallelPVariant=InternalParameters  IdealPVariant=Disabled  IVariant=InternalParameters  DVariant=InternalParameters  IntegratorVariant=Continuous  SatVariant=Disabled  AWVariant=Passthrough  PCopyVariant=Disabled  TRVariant=Disabled  FdbkBlocksVariant=Forward  IdealPFdbkVariant=Disabled  SatFdbkVariant=Disabled  DerivativeFilterVariant=ContFilter  NVariant=InternalParameters  NCopyVariant=Disabled  FilterICVariant=InternalICsFilter  IntegratorICVariant=InternalICs  ExternalResetVariant=Disabled  TRSumVariant=Passthrough  SumFdbkVariant=Disabled  SumVariant=Sum_PID  TsampFilterVariant=InternalTs  TsampNgainVariant=Passthrough  TsampIntegralVariant=Passthrough  ExternalSaturationOutDataTypeStr=Inherit: Same as second input
  Sum : Sum  Inputs=+-|  OutDataTypeStr=double
  Velocity output : Outport
  wires:
  Sum/1 -> PID Controller1/1
  PID Controller1/1 -> Velocity output/1
  Ref/1 -> Sum/1
  Actual Motion/1 -> Sum/2

== system hip_controller_2026_03_03/Subsystem4/PID2 ==
  Ref : Inport
  Actual Motion : Inport  Port=2
  Enable : EnablePort  StatesWhenEnabling=reset
  PID Controller1 : slpidlib/PID Controller  Controller=PID  Form=Parallel  TimeDomain=Continuous-time  UseExternalTs=off  SampleTime=-1  IntegratorMethod=Forward Euler  FilterMethod=Forward Euler  ControllerParametersSource=internal  P=1  I=1  UseKiTs=off  D=0  N=100  UseFilter=on  TunerSelectOption=Transfer Function Based (PID Tuner App)  InitialConditionSource=internal  InitialConditionForIntegrator=0  InitialConditionForFilter=0  DifferentiatorICPrevScaledInput=0  ExternalReset=none  TrackingMode=off  Kt=1  LimitOutput=off  SatLimitsSource=internal  UpperSaturationLimit=inf  LowerSaturationLimit=-inf  LinearizeAsGain=on  AntiWindupMode=none  Kb=1  LimitIntegrator=off  UpperIntegratorSaturationLimit=inf  LowerIntegratorSaturationLimit=-inf  POutMin=[]  POutMax=[]  IOutMin=[]  IOutMax=[]  DOutMin=[]  DOutMax=[]  NOutMin=[]  NOutMax=[]  SumOutMin=[]  SumOutMax=[]  SaturationOutMin=[]  SaturationOutMax=[]  PParamMin=[]  PParamMax=[]  IParamMin=[]  IParamMax=[]  DParamMin=[]  DParamMax=[]  NParamMin=[]  NParamMax=[]  KbParamMin=[]  KbParamMax=[]  KtParamMin=[]  KtParamMax=[]  KbOutMin=[]  KbOutMax=[]  KtOutMin=[]  KtOutMax=[]  IntegratorOutMin=[]  IntegratorOutMax=[]  FilterOutMin=[]  FilterOutMax=[]  SumI1OutMin=[]  SumI1OutMax=[]  SumI2OutMin=[]  SumI2OutMax=[]  SumI3OutMin=[]  SumI3OutMax=[]  SumI4OutMin=[]  SumI4OutMax=[]  SumDOutMin=[]  SumDOutMax=[]  DifferentiatorOutMin=[]  DifferentiatorOutMax=[]  FilterDiffOutCoefMin=[]  FilterDiffOutCoefMax=[]  ReciprocalOutMin=[]  ReciprocalOutMax=[]  SumDenOutMin=[]  SumDenOutMax=[]  SumNumOutMin=[]  SumNumOutMax=[]  DivideOutMin=[]  DivideOutMax=[]  UdiffTsProdOutMin=[]  UdiffTsProdOutMax=[]  NTsProdOutMin=[]  NTsProdOutMax=[]  UintegralTsProdOutMin=[]  UintegralTsProdOutMax=[]  UngainTsProdOutMin=[]  UngainTsProdOutMax=[]  ClampingZeroOutDataTypeStr=Inherit: Inherit via back propagation  ClampingZeroOutMin=[]  ClampingZeroOutMax=[]  FilterDenConstantOutDataTypeStr=Inherit: Inherit via back propagation  FilterDenConstantOutMin=[]  FilterDenConstantOutMax=[]  PCopyOutDataTypeStr=Inherit: Inherit via back propagation  PCopyOutMin=[]  PCopyOutMax=[]  NCopyOutDataTypeStr=Inherit: Inherit via back propagation  NCopyOutMin=[]  NCopyOutMax=[]  IntegratorContinuousStateAttributes=''  IntegratorStateMustResolveToSignalObject=off  IntegratorRTWStateStorageClass=Auto  FilterContinuousStateAttributes=''  FilterStateMustResolveToSignalObject=off  FilterRTWStateStorageClass=Auto  ParallelPVariant=InternalParameters  IdealPVariant=Disabled  IVariant=InternalParameters  DVariant=InternalParameters  IntegratorVariant=Continuous  SatVariant=Disabled  AWVariant=Passthrough  PCopyVariant=Disabled  TRVariant=Disabled  FdbkBlocksVariant=Forward  IdealPFdbkVariant=Disabled  SatFdbkVariant=Disabled  DerivativeFilterVariant=ContFilter  NVariant=InternalParameters  NCopyVariant=Disabled  FilterICVariant=InternalICsFilter  IntegratorICVariant=InternalICs  ExternalResetVariant=Disabled  TRSumVariant=Passthrough  SumFdbkVariant=Disabled  SumVariant=Sum_PID  TsampFilterVariant=InternalTs  TsampNgainVariant=Passthrough  TsampIntegralVariant=Passthrough  ExternalSaturationOutDataTypeStr=Inherit: Same as second input
  Sum : Sum  Inputs=+-|  OutDataTypeStr=double
  Velocity output : Outport
  wires:
  Sum/1 -> PID Controller1/1
  PID Controller1/1 -> Velocity output/1
  Ref/1 -> Sum/1
  Actual Motion/1 -> Sum/2

== system hip_controller_2026_03_03/Subsystem4/PID3 ==
  Ref : Inport
  Actual Motion : Inport  Port=2
  Enable : EnablePort  StatesWhenEnabling=reset
  Gain4 : Gain  Gain=8
  Gain7 : Gain  Gain=0.06-0.04
  Gain8 : Gain  Gain=0
  Integrator1 : Integrator
  Subsystem2 : Subsystem  mask{wn=20, zt=1, x0=0}
      mask prompts: wn "Cut-off frequency (rad/s)"; zt "Damping ratio"; x0 "Initial Condition"
      mask Display: disp('Second-Order\nLow-Pass Filter');
  Sum : Sum  Inputs=|-+  OutDataTypeStr=double
  Sum5 : Sum  Inputs=|+|+|-
  Terminator2 : Terminator
  Velocity output : Outport
  wires:
  Gain7/1 -> Sum5/3
  Subsystem2/2(yd) -> Gain7/1
  Integrator1/1 -> Gain8/1
  Gain4/1 -> Sum5/1
  Actual Motion/1 -> Sum/1
  Gain8/1 -> Sum5/2
  Subsystem2/1(y) -> Terminator2/1
  Sum/1 -> Integrator1/1, Gain4/1
  Ref/1 -> Sum/2
  Sum5/1 -> Velocity output/1, Subsystem2/1(x)

== system hip_controller_2026_03_03/Subsystem4/PID4 ==
  Ref : Inport
  Actual Motion : Inport  Port=2
  Enable : EnablePort  StatesWhenEnabling=reset
  Gain4 : Gain  Gain=8
  Gain7 : Gain  Gain=0.06-0.04
  Gain8 : Gain  Gain=0
  Integrator1 : Integrator
  Subsystem2 : Subsystem  mask{wn=20, zt=1, x0=0}
      mask prompts: wn "Cut-off frequency (rad/s)"; zt "Damping ratio"; x0 "Initial Condition"
      mask Display: disp('Second-Order\nLow-Pass Filter');
  Sum : Sum  Inputs=|-+  OutDataTypeStr=double
  Sum5 : Sum  Inputs=|+|+|-
  Terminator2 : Terminator
  Velocity output : Outport
  wires:
  Gain7/1 -> Sum5/3
  Subsystem2/2(yd) -> Gain7/1
  Integrator1/1 -> Gain8/1
  Gain4/1 -> Sum5/1
  Actual Motion/1 -> Sum/1
  Gain8/1 -> Sum5/2
  Subsystem2/1(y) -> Terminator2/1
  Sum/1 -> Integrator1/1, Gain4/1
  Ref/1 -> Sum/2
  Sum5/1 -> Velocity output/1, Subsystem2/1(x)

== system hip_controller_2026_03_03/Subsystem4/Right Motor Velocity ==
  SWITCH : Inport
  Motor command : Inport  Port=2
  Motor Actual Position Receive : Subsystem
  Subsystem : Subsystem
  MOTOR POSITION : Outport
  MOTOR SPEED : Outport  Port=2
  MOTOR TORQUE : Outport  Port=3
  wires:
  Motor command/1 -> Subsystem/1(Motor command)
  SWITCH/1 -> Motor Actual Position Receive/1(SWITCH), Subsystem/2(SWITCH)
  Motor Actual Position Receive/1(MOTOR POSITION) -> MOTOR POSITION/1
  Motor Actual Position Receive/2(MOTOR SPEED) -> MOTOR SPEED/1
  Motor Actual Position Receive/3(MOTOR TORQUE) -> MOTOR TORQUE/1

== system hip_controller_2026_03_03/Subsystem5/Left Motor Velocity1 ==
  SWITCH : Inport
  Motor command : Inport  Port=2
  Motor Actual Position Receive : Subsystem  Priority=2
  Subsystem : Subsystem  Priority=1
  MOTOR POSITION : Outport
  MOTOR SPEED : Outport  Port=2
  MOTOR TORQUE : Outport  Port=3
  wires:
  Motor command/1 -> Subsystem/1(Motor command)
  SWITCH/1 -> Motor Actual Position Receive/1(SWITCH), Subsystem/2(SWITCH)
  Motor Actual Position Receive/1(MOTOR POSITION) -> MOTOR POSITION/1
  Motor Actual Position Receive/2(MOTOR SPEED) -> MOTOR SPEED/1
  Motor Actual Position Receive/3(MOTOR TORQUE) -> MOTOR TORQUE/1

== system hip_controller_2026_03_03/Subsystem5/PID1 ==
  Ref : Inport
  Actual Motion : Inport  Port=2
  Enable : EnablePort  StatesWhenEnabling=reset
  Gain4 : Gain  Gain=14
  Gain7 : Gain  Gain=0.02
  Gain8 : Gain  Gain=0
  Integrator1 : Integrator
  Subsystem2 : Subsystem  mask{wn=20, zt=1, x0=0}
      mask prompts: wn "Cut-off frequency (rad/s)"; zt "Damping ratio"; x0 "Initial Condition"
      mask Display: disp('Second-Order\nLow-Pass Filter');
  Sum : Sum  Inputs=|-+  OutDataTypeStr=double
  Sum5 : Sum  Inputs=|+|+|-
  Terminator2 : Terminator
  Velocity output : Outport
  wires:
  Gain7/1 -> Sum5/3
  Subsystem2/2(yd) -> Gain7/1
  Integrator1/1 -> Gain8/1
  Gain4/1 -> Sum5/1
  Actual Motion/1 -> Sum/1  "motor_position"
  Gain8/1 -> Sum5/2
  Subsystem2/1(y) -> Terminator2/1
  Sum/1 -> Integrator1/1, Gain4/1
  Ref/1 -> Sum/2  "motor_command"
  Sum5/1 -> Velocity output/1, Subsystem2/1(x)

== system hip_controller_2026_03_03/Subsystem5/PID2 ==
  Ref : Inport
  Actual Motion : Inport  Port=2
  Enable : EnablePort  StatesWhenEnabling=reset
  Gain4 : Gain  Gain=14
  Gain7 : Gain  Gain=0.02
  Gain8 : Gain  Gain=0
  Integrator1 : Integrator
  Subsystem2 : Subsystem  mask{wn=20, zt=1, x0=0}
      mask prompts: wn "Cut-off frequency (rad/s)"; zt "Damping ratio"; x0 "Initial Condition"
      mask Display: disp('Second-Order\nLow-Pass Filter');
  Sum : Sum  Inputs=|-+  OutDataTypeStr=double
  Sum5 : Sum  Inputs=|+|+|-
  Terminator2 : Terminator
  Velocity output : Outport
  wires:
  Gain7/1 -> Sum5/3
  Subsystem2/2(yd) -> Gain7/1
  Integrator1/1 -> Gain8/1
  Gain4/1 -> Sum5/1
  Actual Motion/1 -> Sum/1
  Gain8/1 -> Sum5/2
  Subsystem2/1(y) -> Terminator2/1
  Sum/1 -> Integrator1/1, Gain4/1
  Ref/1 -> Sum/2
  Sum5/1 -> Velocity output/1, Subsystem2/1(x)

== system hip_controller_2026_03_03/Subsystem5/Right Motor Velocity1 ==
  SWITCH : Inport
  Motor command : Inport  Port=2
  Motor Actual Position Receive : Subsystem  Priority=4
  Subsystem : Subsystem  Priority=3
  MOTOR POSITION : Outport
  MOTOR SPEED : Outport  Port=2
  MOTOR TORQUE : Outport  Port=3
  wires:
  Motor command/1 -> Subsystem/1(Motor command)
  SWITCH/1 -> Motor Actual Position Receive/1(SWITCH), Subsystem/2(SWITCH)
  Motor Actual Position Receive/1(MOTOR POSITION) -> MOTOR POSITION/1
  Motor Actual Position Receive/2(MOTOR SPEED) -> MOTOR SPEED/1
  Motor Actual Position Receive/3(MOTOR TORQUE) -> MOTOR TORQUE/1

== system hip_controller_2026_03_03/Subsystem6/Left Motor Velocity ==
  SWITCH : Inport
  Motor command : Inport  Port=2
  Motor Actual Position Receive : Subsystem  Priority=4
  Subsystem : Subsystem  Priority=3
  MOTOR POSITION : Outport
  MOTOR SPEED : Outport  Port=2
  MOTOR TORQUE : Outport  Port=3
  wires:
  Motor command/1 -> Subsystem/1(Motor command)
  SWITCH/1 -> Motor Actual Position Receive/1(SWITCH), Subsystem/2(SWITCH)
  Motor Actual Position Receive/1(MOTOR POSITION) -> MOTOR POSITION/1
  Motor Actual Position Receive/2(MOTOR SPEED) -> MOTOR SPEED/1
  Motor Actual Position Receive/3(MOTOR TORQUE) -> MOTOR TORQUE/1

== system hip_controller_2026_03_03/Subsystem6/Right Motor Velocity ==
  SWITCH : Inport
  Motor command : Inport  Port=2
  Motor Actual Position Receive : Subsystem  Priority=2
  Subsystem : Subsystem  Priority=1
  MOTOR POSITION : Outport
  MOTOR SPEED : Outport  Port=2
  MOTOR TORQUE : Outport  Port=3
  wires:
  Motor command/1 -> Subsystem/1(Motor command)
  SWITCH/1 -> Motor Actual Position Receive/1(SWITCH), Subsystem/2(SWITCH)
  Motor Actual Position Receive/1(MOTOR POSITION) -> MOTOR POSITION/1
  Motor Actual Position Receive/2(MOTOR SPEED) -> MOTOR SPEED/1
  Motor Actual Position Receive/3(MOTOR TORQUE) -> MOTOR TORQUE/1

== system hip_controller_2026_03_03/Subsystem6/Subsystem1 ==
  x : Inport
  Constant : Constant  Value=2
  Integrator1 : Integrator  InitialConditionSource=external
  Integrator2 : Integrator
  Product : Product  RndMeth=Zero
  Product1 : Product  RndMeth=Zero
  Product2 : Product  Inputs=3  RndMeth=Zero
  Sum : Sum  Inputs=|+-
  Sum1 : Sum  Inputs=|+-
  wn : Constant  Value=wn
  x0 : Constant  Value=x0
  zt : Constant  Value=zt
  y : Outport  VectorParamsAs1DForOutWhenUnconnected=off
  yd : Outport  Port=2  VectorParamsAs1DForOutWhenUnconnected=off
  wires:
  Sum/1 -> Product/2
  wn/1 -> Product/1, Product1/1
  Sum1/1 -> Sum/1
  x0/1 -> Integrator1/2
  Integrator2/1 -> Product1/2, Product2/1
  Product/1 -> Integrator2/1
  x/1 -> Sum1/1
  Product1/1 -> Integrator1/1, yd/1
  Integrator1/1 -> Sum1/2, y/1
  Product2/1 -> Sum/2
  zt/1 -> Product2/3
  Constant/1 -> Product2/2

== system hip_controller_2026_03_03/Subsystem6/Subsystem4 ==
  x : Inport
  Constant : Constant  Value=2
  Integrator1 : Integrator  InitialConditionSource=external
  Integrator2 : Integrator
  Product : Product  RndMeth=Zero
  Product1 : Product  RndMeth=Zero
  Product2 : Product  Inputs=3  RndMeth=Zero
  Sum : Sum  Inputs=|+-
  Sum1 : Sum  Inputs=|+-
  wn : Constant  Value=wn
  x0 : Constant  Value=x0
  zt : Constant  Value=zt
  y : Outport  VectorParamsAs1DForOutWhenUnconnected=off
  yd : Outport  Port=2  VectorParamsAs1DForOutWhenUnconnected=off
  wires:
  Sum/1 -> Product/2
  wn/1 -> Product/1, Product1/1
  Sum1/1 -> Sum/1
  x0/1 -> Integrator1/2
  Integrator2/1 -> Product1/2, Product2/1
  Product/1 -> Integrator2/1
  x/1 -> Sum1/1
  Product1/1 -> Integrator1/1, yd/1
  Integrator1/1 -> Sum1/2, y/1
  Product2/1 -> Sum/2
  zt/1 -> Product2/3
  Constant/1 -> Product2/2

== system hip_controller_2026_03_03/Initialize Function/Config_L /Enter Config Mode ==
  Compare To Zero8 : simulink/Logic and Bit Operations/Compare To Zero  relop===  OutDataTypeStr=boolean
  Constant5 : Constant  Value=0x00
  Start_Config_L : arduinolib/I2C Write  I2CModule=0  Mode=Master  SlaveAddress=0x28  SlaveByteOrder=BigEndian  Direction=Transmitter  RegisterAddressMode=on  RegisterAddress=0x3D  SlaveDataType=uint8  DataLength=1  NoAck=off  RepeatedStart=off  OutputStatus=on  blockPlatform=ARDUINO
      settings: SourceProductName=Common
  Status : Outport
  wires:
  Start_Config_L/1 -> Compare To Zero8/1  "0 for success"
  Constant5/1 -> Start_Config_L/1
  Compare To Zero8/1 -> Status/1

== system hip_controller_2026_03_03/Initialize Function/Config_L /Start Fused (NDOF) Mode ==
  Enable : EnablePort
  Compare To Constant2 : simulink/Logic and Bit Operations/Compare To Constant  relop===  const=0  OutDataTypeStr=boolean
  Constant4 : Constant  Value=0x0C
  I2C Write8 : arduinolib/I2C Write  I2CModule=0  Mode=Master  SlaveAddress=0x28  SlaveByteOrder=BigEndian  Direction=Transmitter  RegisterAddressMode=on  RegisterAddress=0x3D  SlaveDataType=uint8  DataLength=1  NoAck=off  RepeatedStart=off  OutputStatus=on  blockPlatform=ARDUINO
      settings: SourceProductName=Common
  Status : Outport
  wires:
  Compare To Constant2/1 -> Status/1
  Constant4/1 -> I2C Write8/1
  I2C Write8/1 -> Compare To Constant2/1  "0: success"

== system hip_controller_2026_03_03/Initialize Function/Config_L /X=Z, Y=Y, Z=X ==
  Enable : EnablePort
  Compare To Constant : simulink/Logic and Bit Operations/Compare To Constant  relop=~=  const=hex2dec('06')  OutDataTypeStr=boolean
  Compare To Constant1 : simulink/Logic and Bit Operations/Compare To Constant  relop===  const=hex2dec('06')  OutDataTypeStr=boolean
  Enabled Subsystem : Subsystem  TreatAsAtomicUnit=on
  I2C Read : arduinolib/I2C Read  I2CModule=0  Mode=Master  SlaveAddress=0x28  SlaveByteOrder=LittleEndian  Direction=Receiver  RegisterAddressMode=on  RegisterAddress=0x41  SlaveDataType=uint8  DataLength=1  NoAck=off  RepeatedStart=off  OutputStatus=off  blockPlatform=ARDUINO  SampleTime=-1
      settings: SourceProductName=Common
  OR : Logic  Operator=OR  IconShape=distinctive  AllPortsSameDT=off  OutDataTypeStr=boolean
  Status : Outport
  wires:
  I2C Read/1 -> Compare To Constant1/1, Compare To Constant/1
  Compare To Constant1/1 -> OR/2
  Compare To Constant/1 -> Enabled Subsystem/Enable
  Enabled Subsystem/1(Status) -> OR/1
  OR/1 -> Status/1
